simulink model "c00023M_harness"  (R2018a)
settings: Solver=ode3  StartTime=0.0  StopTime=10.0  RelTol=1e-3  EnableMultiTasking=on
undefined symbols (not defined in the file): b, DiscIntNeverNeededParam, J, K, L, PosMinimaW3, PosMinimaW4, R, sigbuilder_block
(part 22 of 72)

== system c00023M_harness/M154/S3 ==
  PhyMeasure : Inport
  SensorOut : Outport
  wires:
  PhyMeasure/1 -> SensorOut/1

== system c00023M_harness/M154/S4 ==
  PhyMeasure : Inport
  SensorOut : Outport
  wires:
  PhyMeasure/1 -> SensorOut/1

== system c00023M_harness/M155/Cyber ==
  note: Sensors
  note: Inputs For Window1
  note: Inputs for Window 2
  note: Inputs for window 3
  note: Inputs for window 4
  note: Users
  note: Users
  note: Sensors
  note: Users
  note: Sensors
  note: Users
  note: Sensors
  note: USERS
      | ---------------------------------
      | 0: None
      | 1: Ventana Arriba
      | 2: Ventana hasta arriba
      | 3: Ventana abajo
      | 4: Ventana hasta abajo
  note: 1: SUBE
      | 0: PARADO
      | -1 BAJA
  note: D = Driver (W1)
      | P1 = Passenger 1 (W2)
      | P2 = Passenger 2 (W3)
      | P3 = Passenger 3 (W4)
      | O = Obstacle
      | C = Control
      | Pri = Prioritizer
      | LD = LockDriver
      | PosW = PositionWindow
      | WL = WindowLogic
      | OW = ObstacleWindow
      | CWXC = ControlWindowXCentralized
      | S = Sensor
      | L = Lock
      | WPos = WindowPosition
      | M = Memory
      | InW = InputWindow
      | WIn = WindowInput
  PosW1 : Inport
  PosW2 : Inport  Port=2
  PosW3 : Inport  Port=3
  PosW4 : Inport  Port=4
  DW1 : Inport  Port=5
  DW3 : Inport  Port=6
  P1W2 : Inport  Port=7
  P2W3 : Inport  Port=8
  P3W4 : Inport  Port=9
  P1W4 : Inport  Port=10
  OW1 : Inport  Port=11
  OW2 : Inport  Port=12
  OW3 : Inport  Port=13
  OW4 : Inport  Port=14
  LD : Inport  Port=15
  CW3C : Inport  Port=16
  CW4C : Inport  Port=17
  Pri1 : Subsystem
  Pri4 : Subsystem
  WL : Subsystem
  WL1 : Subsystem
  WL2 : Subsystem
  WL3 : Subsystem
  W1 : Outport
  W2 : Outport  Port=2
  W3 : Outport  Port=3
  W4 : Outport  Port=4
  wires:
  CW4C/1 -> Pri4/3(CW4C)
  CW3C/1 -> Pri1/3(CW3C)
  WL3/1(WindowLogicOutput) -> W4/1
  WL2/1(WindowLogicOutput) -> W3/1
  Pri4/1(User) -> WL3/2(User)
  OW4/1 -> WL3/3(OW)
  PosW4/1 -> WL3/1(WPos)
  P1W4/1 -> Pri4/2(P1)
  P3W4/1 -> Pri4/1(P)
  P2W3/1 -> Pri1/2(P)
  DW3/1 -> Pri1/1(D)
  OW3/1 -> WL2/3(OW)
  PosW3/1 -> WL2/1(WPos)
  Pri1/1(User) -> WL2/2(User)
  WL1/1(WindowLogicOutput) -> W2/1
  OW2/1 -> WL1/3(OW)
  PosW2/1 -> WL1/1(WPos)
  WL/1(WindowLogicOutput) -> W1/1
  OW1/1 -> WL/3(OW)
  PosW1/1 -> WL/1(WPos)
  LD/1 -> WL2/4(L), WL3/4(L)
  DW1/1 -> WL/2(User)
  P1W2/1 -> WL1/2(User)

== system c00023M_harness/M155/Physical ==
  InW1 : Inport
  InW2 : Inport  Port=2
  InW3 : Inport  Port=3
  InW4 : Inport  Port=4
  W : Subsystem
  W5 : Subsystem
  W6 : Subsystem
  W7 : Subsystem
  W1 : Outport
  W2 : Outport  Port=2
  W3 : Outport  Port=3
  W4 : Outport  Port=4
  wires:
  W7/1(WPos) -> W4/1
  W6/1(WPos) -> W3/1
  W5/1(WPos) -> W2/1
  W/1(WPos) -> W1/1
  InW4/1 -> W7/1(WIn)
  InW3/1 -> W6/1(WIn)
  InW2/1 -> W5/1(WIn)
  InW1/1 -> W/1(WIn)

== system c00023M_harness/M155/S1 ==
  PhyMeasure : Inport
  SensorOut : Outport
  wires:
  PhyMeasure/1 -> SensorOut/1

== system c00023M_harness/M155/S2 ==
  PhyMeasure : Inport
  SensorOut : Outport
  wires:
  PhyMeasure/1 -> SensorOut/1

== system c00023M_harness/M155/S3 ==
  PhyMeasure : Inport
  SensorOut : Outport
  wires:
  PhyMeasure/1 -> SensorOut/1

== system c00023M_harness/M155/S4 ==
  PhyMeasure : Inport
  SensorOut : Outport
  wires:
  PhyMeasure/1 -> SensorOut/1

== system c00023M_harness/M156/Cyber ==
  note: Sensors
  note: Inputs For Window1
  note: Inputs for Window 2
  note: Inputs for window 3
  note: Inputs for window 4
  note: Users
  note: Users
  note: Sensors
  note: Users
  note: Sensors
  note: Users
  note: Sensors
  note: USERS
      | ---------------------------------
      | 0: None
      | 1: Ventana Arriba
      | 2: Ventana hasta arriba
      | 3: Ventana abajo
      | 4: Ventana hasta abajo
  note: 1: SUBE
      | 0: PARADO
      | -1 BAJA
  note: D = Driver (W1)
      | P1 = Passenger 1 (W2)
      | P2 = Passenger 2 (W3)
      | P3 = Passenger 3 (W4)
      | O = Obstacle
      | C = Control
      | Pri = Prioritizer
      | LD = LockDriver
      | PosW = PositionWindow
      | WL = WindowLogic
      | OW = ObstacleWindow
      | CWXC = ControlWindowXCentralized
      | S = Sensor
      | L = Lock
      | WPos = WindowPosition
      | M = Memory
      | InW = InputWindow
      | WIn = WindowInput
  PosW1 : Inport
  PosW2 : Inport  Port=2
  PosW3 : Inport  Port=3
  PosW4 : Inport  Port=4
  DW1 : Inport  Port=5
  DW3 : Inport  Port=6
  P1W2 : Inport  Port=7
  P2W3 : Inport  Port=8
  P3W4 : Inport  Port=9
  P1W4 : Inport  Port=10
  OW1 : Inport  Port=11
  OW2 : Inport  Port=12
  OW3 : Inport  Port=13
  OW4 : Inport  Port=14
  LD : Inport  Port=15
  CW3C : Inport  Port=16
  CW4C : Inport  Port=17
  Pri1 : Subsystem
  Pri4 : Subsystem
  WL : Subsystem
  WL1 : Subsystem
  WL2 : Subsystem
  WL3 : Subsystem
  W1 : Outport
  W2 : Outport  Port=2
  W3 : Outport  Port=3
  W4 : Outport  Port=4
  wires:
  CW4C/1 -> Pri4/3(CW4C)
  CW3C/1 -> Pri1/3(CW3C)
  WL3/1(WindowLogicOutput) -> W4/1
  WL2/1(WindowLogicOutput) -> W3/1
  Pri4/1(User) -> WL3/2(User)
  OW4/1 -> WL3/3(OW)
  PosW4/1 -> WL3/1(WPos)
  P1W4/1 -> Pri4/2(P1)
  P3W4/1 -> Pri4/1(P)
  P2W3/1 -> Pri1/2(P)
  DW3/1 -> Pri1/1(D)
  OW3/1 -> WL2/3(OW)
  PosW3/1 -> WL2/1(WPos)
  Pri1/1(User) -> WL2/2(User)
  WL1/1(WindowLogicOutput) -> W2/1
  OW2/1 -> WL1/3(OW)
  PosW2/1 -> WL1/1(WPos)
  WL/1(WindowLogicOutput) -> W1/1
  OW1/1 -> WL/3(OW)
  PosW1/1 -> WL/1(WPos)
  LD/1 -> WL2/4(L), WL3/4(L)
  DW1/1 -> WL/2(User)
  P1W2/1 -> WL1/2(User)

== system c00023M_harness/M156/Physical ==
  InW1 : Inport
  InW2 : Inport  Port=2
  InW3 : Inport  Port=3
  InW4 : Inport  Port=4
  W : Subsystem
  W5 : Subsystem
  W6 : Subsystem
  W7 : Subsystem
  W1 : Outport
  W2 : Outport  Port=2
  W3 : Outport  Port=3
  W4 : Outport  Port=4
  wires:
  W7/1(WPos) -> W4/1
  W6/1(WPos) -> W3/1
  W5/1(WPos) -> W2/1
  W/1(WPos) -> W1/1
  InW4/1 -> W7/1(WIn)
  InW3/1 -> W6/1(WIn)
  InW2/1 -> W5/1(WIn)
  InW1/1 -> W/1(WIn)

== system c00023M_harness/M156/S1 ==
  PhyMeasure : Inport
  SensorOut : Outport
  wires:
  PhyMeasure/1 -> SensorOut/1

== system c00023M_harness/M156/S2 ==
  PhyMeasure : Inport
  SensorOut : Outport
  wires:
  PhyMeasure/1 -> SensorOut/1

== system c00023M_harness/M156/S3 ==
  PhyMeasure : Inport
  SensorOut : Outport
  wires:
  PhyMeasure/1 -> SensorOut/1

== system c00023M_harness/M156/S4 ==
  PhyMeasure : Inport
  SensorOut : Outport
  wires:
  PhyMeasure/1 -> SensorOut/1

== system c00023M_harness/M157/Cyber ==
  note: Sensors
  note: Inputs For Window1
  note: Inputs for Window 2
  note: Inputs for window 3
  note: Inputs for window 4
  note: Users
  note: Users
  note: Sensors
  note: Users
  note: Sensors
  note: Users
  note: Sensors
  note: USERS
      | ---------------------------------
      | 0: None
      | 1: Ventana Arriba
      | 2: Ventana hasta arriba
      | 3: Ventana abajo
      | 4: Ventana hasta abajo
  note: 1: SUBE
      | 0: PARADO
      | -1 BAJA
  note: D = Driver (W1)
      | P1 = Passenger 1 (W2)
      | P2 = Passenger 2 (W3)
      | P3 = Passenger 3 (W4)
      | O = Obstacle
      | C = Control
      | Pri = Prioritizer
      | LD = LockDriver
      | PosW = PositionWindow
      | WL = WindowLogic
      | OW = ObstacleWindow
      | CWXC = ControlWindowXCentralized
      | S = Sensor
      | L = Lock
      | WPos = WindowPosition
      | M = Memory
      | InW = InputWindow
      | WIn = WindowInput
  PosW1 : Inport
  PosW2 : Inport  Port=2
  PosW3 : Inport  Port=3
  PosW4 : Inport  Port=4
  DW1 : Inport  Port=5
  DW3 : Inport  Port=6
  P1W2 : Inport  Port=7
  P2W3 : Inport  Port=8
  P3W4 : Inport  Port=9
  P1W4 : Inport  Port=10
  OW1 : Inport  Port=11
  OW2 : Inport  Port=12
  OW3 : Inport  Port=13
  OW4 : Inport  Port=14
  LD : Inport  Port=15
  CW3C : Inport  Port=16
  CW4C : Inport  Port=17
  Pri1 : Subsystem
  Pri4 : Subsystem
  WL : Subsystem
  WL1 : Subsystem
  WL2 : Subsystem
  WL3 : Subsystem
  W1 : Outport
  W2 : Outport  Port=2
  W3 : Outport  Port=3
  W4 : Outport  Port=4
  wires:
  CW4C/1 -> Pri4/3(CW4C)
  CW3C/1 -> Pri1/3(CW3C)
  WL3/1(WindowLogicOutput) -> W4/1
  WL2/1(WindowLogicOutput) -> W3/1
  Pri4/1(User) -> WL3/2(User)
  OW4/1 -> WL3/3(OW)
  PosW4/1 -> WL3/1(WPos)
  P1W4/1 -> Pri4/2(P1)
  P3W4/1 -> Pri4/1(P)
  P2W3/1 -> Pri1/2(P)
  DW3/1 -> Pri1/1(D)
  OW3/1 -> WL2/3(OW)
  PosW3/1 -> WL2/1(WPos)
  Pri1/1(User) -> WL2/2(User)
  WL1/1(WindowLogicOutput) -> W2/1
  OW2/1 -> WL1/3(OW)
  PosW2/1 -> WL1/1(WPos)
  WL/1(WindowLogicOutput) -> W1/1
  OW1/1 -> WL/3(OW)
  PosW1/1 -> WL/1(WPos)
  LD/1 -> WL2/4(L), WL3/4(L)
  DW1/1 -> WL/2(User)
  P1W2/1 -> WL1/2(User)

== system c00023M_harness/M157/Physical ==
  InW1 : Inport
  InW2 : Inport  Port=2
  InW3 : Inport  Port=3
  InW4 : Inport  Port=4
  W : Subsystem
  W5 : Subsystem
  W6 : Subsystem
  W7 : Subsystem
  W1 : Outport
  W2 : Outport  Port=2
  W3 : Outport  Port=3
  W4 : Outport  Port=4
  wires:
  W7/1(WPos) -> W4/1
  W6/1(WPos) -> W3/1
  W5/1(WPos) -> W2/1
  W/1(WPos) -> W1/1
  InW4/1 -> W7/1(WIn)
  InW3/1 -> W6/1(WIn)
  InW2/1 -> W5/1(WIn)
  InW1/1 -> W/1(WIn)

== system c00023M_harness/M157/S1 ==
  PhyMeasure : Inport
  SensorOut : Outport
  wires:
  PhyMeasure/1 -> SensorOut/1

== system c00023M_harness/M157/S2 ==
  PhyMeasure : Inport
  SensorOut : Outport
  wires:
  PhyMeasure/1 -> SensorOut/1

== system c00023M_harness/M157/S3 ==
  PhyMeasure : Inport
  SensorOut : Outport
  wires:
  PhyMeasure/1 -> SensorOut/1

== system c00023M_harness/M157/S4 ==
  PhyMeasure : Inport
  SensorOut : Outport
  wires:
  PhyMeasure/1 -> SensorOut/1

== system c00023M_harness/M158/Cyber ==
  note: Sensors
  note: Inputs For Window1
  note: Inputs for Window 2
  note: Inputs for window 3
  note: Inputs for window 4
  note: Users
  note: Users
  note: Sensors
  note: Users
  note: Sensors
  note: Users
  note: Sensors
  note: USERS
      | ---------------------------------
      | 0: None
      | 1: Ventana Arriba
      | 2: Ventana hasta arriba
      | 3: Ventana abajo
      | 4: Ventana hasta abajo
  note: 1: SUBE
      | 0: PARADO
      | -1 BAJA
  note: D = Driver (W1)
      | P1 = Passenger 1 (W2)
      | P2 = Passenger 2 (W3)
      | P3 = Passenger 3 (W4)
      | O = Obstacle
      | C = Control
      | Pri = Prioritizer
      | LD = LockDriver
      | PosW = PositionWindow
      | WL = WindowLogic
      | OW = ObstacleWindow
      | CWXC = ControlWindowXCentralized
      | S = Sensor
      | L = Lock
      | WPos = WindowPosition
      | M = Memory
      | InW = InputWindow
      | WIn = WindowInput
  PosW1 : Inport
  PosW2 : Inport  Port=2
  PosW3 : Inport  Port=3
  PosW4 : Inport  Port=4
  DW1 : Inport  Port=5
  DW3 : Inport  Port=6
  P1W2 : Inport  Port=7
  P2W3 : Inport  Port=8
  P3W4 : Inport  Port=9
  P1W4 : Inport  Port=10
  OW1 : Inport  Port=11
  OW2 : Inport  Port=12
  OW3 : Inport  Port=13
  OW4 : Inport  Port=14
  LD : Inport  Port=15
  CW3C : Inport  Port=16
  CW4C : Inport  Port=17
  Pri1 : Subsystem
  Pri4 : Subsystem
  WL : Subsystem
  WL1 : Subsystem
  WL2 : Subsystem
  WL3 : Subsystem
  W1 : Outport
  W2 : Outport  Port=2
  W3 : Outport  Port=3
  W4 : Outport  Port=4
  wires:
  CW4C/1 -> Pri4/3(CW4C)
  CW3C/1 -> Pri1/3(CW3C)
  WL3/1(WindowLogicOutput) -> W4/1
  WL2/1(WindowLogicOutput) -> W3/1
  Pri4/1(User) -> WL3/2(User)
  OW4/1 -> WL3/3(OW)
  PosW4/1 -> WL3/1(WPos)
  P1W4/1 -> Pri4/2(P1)
  P3W4/1 -> Pri4/1(P)
  P2W3/1 -> Pri1/2(P)
  DW3/1 -> Pri1/1(D)
  OW3/1 -> WL2/3(OW)
  PosW3/1 -> WL2/1(WPos)
  Pri1/1(User) -> WL2/2(User)
  WL1/1(WindowLogicOutput) -> W2/1
  OW2/1 -> WL1/3(OW)
  PosW2/1 -> WL1/1(WPos)
  WL/1(WindowLogicOutput) -> W1/1
  OW1/1 -> WL/3(OW)
  PosW1/1 -> WL/1(WPos)
  LD/1 -> WL2/4(L), WL3/4(L)
  DW1/1 -> WL/2(User)
  P1W2/1 -> WL1/2(User)

== system c00023M_harness/M158/Physical ==
  InW1 : Inport
  InW2 : Inport  Port=2
  InW3 : Inport  Port=3
  InW4 : Inport  Port=4
  W : Subsystem
  W5 : Subsystem
  W6 : Subsystem
  W7 : Subsystem
  W1 : Outport
  W2 : Outport  Port=2
  W3 : Outport  Port=3
  W4 : Outport  Port=4
  wires:
  W7/1(WPos) -> W4/1
  W6/1(WPos) -> W3/1
  W5/1(WPos) -> W2/1
  W/1(WPos) -> W1/1
  InW4/1 -> W7/1(WIn)
  InW3/1 -> W6/1(WIn)
  InW2/1 -> W5/1(WIn)
  InW1/1 -> W/1(WIn)

== system c00023M_harness/M158/S1 ==
  PhyMeasure : Inport
  SensorOut : Outport
  wires:
  PhyMeasure/1 -> SensorOut/1

== system c00023M_harness/M158/S2 ==
  PhyMeasure : Inport
  SensorOut : Outport
  wires:
  PhyMeasure/1 -> SensorOut/1

== system c00023M_harness/M158/S3 ==
  PhyMeasure : Inport
  SensorOut : Outport
  wires:
  PhyMeasure/1 -> SensorOut/1

== system c00023M_harness/M158/S4 ==
  PhyMeasure : Inport
  SensorOut : Outport
  wires:
  PhyMeasure/1 -> SensorOut/1

== system c00023M_harness/M159/Cyber ==
  note: Sensors
  note: Inputs For Window1
  note: Inputs for Window 2
  note: Inputs for window 3
  note: Inputs for window 4
  note: Users
  note: Users
  note: Sensors
  note: Users
  note: Sensors
  note: Users
  note: Sensors
  note: USERS
      | ---------------------------------
      | 0: None
      | 1: Ventana Arriba
      | 2: Ventana hasta arriba
      | 3: Ventana abajo
      | 4: Ventana hasta abajo
  note: 1: SUBE
      | 0: PARADO
      | -1 BAJA
  note: D = Driver (W1)
      | P1 = Passenger 1 (W2)
      | P2 = Passenger 2 (W3)
      | P3 = Passenger 3 (W4)
      | O = Obstacle
      | C = Control
      | Pri = Prioritizer
      | LD = LockDriver
      | PosW = PositionWindow
      | WL = WindowLogic
      | OW = ObstacleWindow
      | CWXC = ControlWindowXCentralized
      | S = Sensor
      | L = Lock
      | WPos = WindowPosition
      | M = Memory
      | InW = InputWindow
      | WIn = WindowInput
  PosW1 : Inport
  PosW2 : Inport  Port=2
  PosW3 : Inport  Port=3
  PosW4 : Inport  Port=4
  DW1 : Inport  Port=5
  DW3 : Inport  Port=6
  P1W2 : Inport  Port=7
  P2W3 : Inport  Port=8
  P3W4 : Inport  Port=9
  P1W4 : Inport  Port=10
  OW1 : Inport  Port=11
  OW2 : Inport  Port=12
  OW3 : Inport  Port=13
  OW4 : Inport  Port=14
  LD : Inport  Port=15
  CW3C : Inport  Port=16
  CW4C : Inport  Port=17
  Pri1 : Subsystem
  Pri4 : Subsystem
  WL : Subsystem
  WL1 : Subsystem
  WL2 : Subsystem
  WL3 : Subsystem
  W1 : Outport
  W2 : Outport  Port=2
  W3 : Outport  Port=3
  W4 : Outport  Port=4
  wires:
  CW4C/1 -> Pri4/3(CW4C)
  CW3C/1 -> Pri1/3(CW3C)
  WL3/1(WindowLogicOutput) -> W4/1
  WL2/1(WindowLogicOutput) -> W3/1
  Pri4/1(User) -> WL3/2(User)
  OW4/1 -> WL3/3(OW)
  PosW4/1 -> WL3/1(WPos)
  P1W4/1 -> Pri4/2(P1)
  P3W4/1 -> Pri4/1(P)
  P2W3/1 -> Pri1/2(P)
  DW3/1 -> Pri1/1(D)
  OW3/1 -> WL2/3(OW)
  PosW3/1 -> WL2/1(WPos)
  Pri1/1(User) -> WL2/2(User)
  WL1/1(WindowLogicOutput) -> W2/1
  OW2/1 -> WL1/3(OW)
  PosW2/1 -> WL1/1(WPos)
  WL/1(WindowLogicOutput) -> W1/1
  OW1/1 -> WL/3(OW)
  PosW1/1 -> WL/1(WPos)
  LD/1 -> WL2/4(L), WL3/4(L)
  DW1/1 -> WL/2(User)
  P1W2/1 -> WL1/2(User)

== system c00023M_harness/M159/Physical ==
  InW1 : Inport
  InW2 : Inport  Port=2
  InW3 : Inport  Port=3
  InW4 : Inport  Port=4
  W : Subsystem
  W5 : Subsystem
  W6 : Subsystem
  W7 : Subsystem
  W1 : Outport
  W2 : Outport  Port=2
  W3 : Outport  Port=3
  W4 : Outport  Port=4
  wires:
  W7/1(WPos) -> W4/1
  W6/1(WPos) -> W3/1
  W5/1(WPos) -> W2/1
  W/1(WPos) -> W1/1
  InW4/1 -> W7/1(WIn)
  InW3/1 -> W6/1(WIn)
  InW2/1 -> W5/1(WIn)
  InW1/1 -> W/1(WIn)

== system c00023M_harness/M159/S1 ==
  PhyMeasure : Inport
  SensorOut : Outport
  wires:
  PhyMeasure/1 -> SensorOut/1

== system c00023M_harness/M159/S2 ==
  PhyMeasure : Inport
  SensorOut : Outport
  wires:
  PhyMeasure/1 -> SensorOut/1

== system c00023M_harness/M159/S3 ==
  PhyMeasure : Inport
  SensorOut : Outport
  wires:
  PhyMeasure/1 -> SensorOut/1

== system c00023M_harness/M159/S4 ==
  PhyMeasure : Inport
  SensorOut : Outport
  wires:
  PhyMeasure/1 -> SensorOut/1

== system c00023M_harness/M160/Cyber ==
  note: Sensors
  note: Inputs For Window1
  note: Inputs for Window 2
  note: Inputs for window 3
  note: Inputs for window 4
  note: Users
  note: Users
  note: Sensors
  note: Users
  note: Sensors
  note: Users
  note: Sensors
  note: USERS
      | ---------------------------------
      | 0: None
      | 1: Ventana Arriba
      | 2: Ventana hasta arriba
      | 3: Ventana abajo
      | 4: Ventana hasta abajo
  note: 1: SUBE
      | 0: PARADO
      | -1 BAJA
  note: D = Driver (W1)
      | P1 = Passenger 1 (W2)
      | P2 = Passenger 2 (W3)
      | P3 = Passenger 3 (W4)
      | O = Obstacle
      | C = Control
      | Pri = Prioritizer
      | LD = LockDriver
      | PosW = PositionWindow
      | WL = WindowLogic
      | OW = ObstacleWindow
      | CWXC = ControlWindowXCentralized
      | S = Sensor
      | L = Lock
      | WPos = WindowPosition
      | M = Memory
      | InW = InputWindow
      | WIn = WindowInput
  PosW1 : Inport
  PosW2 : Inport  Port=2
  PosW3 : Inport  Port=3
  PosW4 : Inport  Port=4
  DW1 : Inport  Port=5
  DW3 : Inport  Port=6
  P1W2 : Inport  Port=7
  P2W3 : Inport  Port=8
  P3W4 : Inport  Port=9
  P1W4 : Inport  Port=10
  OW1 : Inport  Port=11
  OW2 : Inport  Port=12
  OW3 : Inport  Port=13
  OW4 : Inport  Port=14
  LD : Inport  Port=15
  CW3C : Inport  Port=16
  CW4C : Inport  Port=17
  Pri1 : Subsystem
  Pri4 : Subsystem
  WL : Subsystem
  WL1 : Subsystem
  WL2 : Subsystem
  WL3 : Subsystem
  W1 : Outport
  W2 : Outport  Port=2
  W3 : Outport  Port=3
  W4 : Outport  Port=4
  wires:
  CW4C/1 -> Pri4/3(CW4C)
  CW3C/1 -> Pri1/3(CW3C)
  WL3/1(WindowLogicOutput) -> W4/1
  WL2/1(WindowLogicOutput) -> W3/1
  Pri4/1(User) -> WL3/2(User)
  OW4/1 -> WL3/3(OW)
  PosW4/1 -> WL3/1(WPos)
  P1W4/1 -> Pri4/2(P1)
  P3W4/1 -> Pri4/1(P)
  P2W3/1 -> Pri1/2(P)
  DW3/1 -> Pri1/1(D)
  OW3/1 -> WL2/3(OW)
  PosW3/1 -> WL2/1(WPos)
  Pri1/1(User) -> WL2/2(User)
  WL1/1(WindowLogicOutput) -> W2/1
  OW2/1 -> WL1/3(OW)
  PosW2/1 -> WL1/1(WPos)
  WL/1(WindowLogicOutput) -> W1/1
  OW1/1 -> WL/3(OW)
  PosW1/1 -> WL/1(WPos)
  LD/1 -> WL2/4(L), WL3/4(L)
  DW1/1 -> WL/2(User)
  P1W2/1 -> WL1/2(User)

== system c00023M_harness/M160/Physical ==
  InW1 : Inport
  InW2 : Inport  Port=2
  InW3 : Inport  Port=3
  InW4 : Inport  Port=4
  W : Subsystem
  W5 : Subsystem
  W6 : Subsystem
  W7 : Subsystem
  W1 : Outport
  W2 : Outport  Port=2
  W3 : Outport  Port=3
  W4 : Outport  Port=4
  wires:
  W7/1(WPos) -> W4/1
  W6/1(WPos) -> W3/1
  W5/1(WPos) -> W2/1
  W/1(WPos) -> W1/1
  InW4/1 -> W7/1(WIn)
  InW3/1 -> W6/1(WIn)
  InW2/1 -> W5/1(WIn)
  InW1/1 -> W/1(WIn)

== system c00023M_harness/M160/S1 ==
  PhyMeasure : Inport
  SensorOut : Outport
  wires:
  PhyMeasure/1 -> SensorOut/1

== system c00023M_harness/M160/S2 ==
  PhyMeasure : Inport
  SensorOut : Outport
  wires:
  PhyMeasure/1 -> SensorOut/1

== system c00023M_harness/M160/S3 ==
  PhyMeasure : Inport
  SensorOut : Outport
  wires:
  PhyMeasure/1 -> SensorOut/1

== system c00023M_harness/M160/S4 ==
  PhyMeasure : Inport
  SensorOut : Outport
  wires:
  PhyMeasure/1 -> SensorOut/1

== system c00023M_harness/M161/Cyber ==
  note: Sensors
  note: Inputs For Window1
  note: Inputs for Window 2
  note: Inputs for window 3
  note: Inputs for window 4
  note: Users
  note: Users
  note: Sensors
  note: Users
  note: Sensors
  note: Users
  note: Sensors
  note: USERS
      | ---------------------------------
      | 0: None
      | 1: Ventana Arriba
      | 2: Ventana hasta arriba
      | 3: Ventana abajo
      | 4: Ventana hasta abajo
  note: 1: SUBE
      | 0: PARADO
      | -1 BAJA
  note: D = Driver (W1)
      | P1 = Passenger 1 (W2)
      | P2 = Passenger 2 (W3)
      | P3 = Passenger 3 (W4)
      | O = Obstacle
      | C = Control
      | Pri = Prioritizer
      | LD = LockDriver
      | PosW = PositionWindow
      | WL = WindowLogic
      | OW = ObstacleWindow
      | CWXC = ControlWindowXCentralized
      | S = Sensor
      | L = Lock
      | WPos = WindowPosition
      | M = Memory
      | InW = InputWindow
      | WIn = WindowInput
  PosW1 : Inport
  PosW2 : Inport  Port=2
  PosW3 : Inport  Port=3
  PosW4 : Inport  Port=4
  DW1 : Inport  Port=5
  DW3 : Inport  Port=6
  P1W2 : Inport  Port=7
  P2W3 : Inport  Port=8
  P3W4 : Inport  Port=9
  P1W4 : Inport  Port=10
  OW1 : Inport  Port=11
  OW2 : Inport  Port=12
  OW3 : Inport  Port=13
  OW4 : Inport  Port=14
  LD : Inport  Port=15
  CW3C : Inport  Port=16
  CW4C : Inport  Port=17
  Pri1 : Subsystem
  Pri4 : Subsystem
  WL : Subsystem
  WL1 : Subsystem
  WL2 : Subsystem
  WL3 : Subsystem
  W1 : Outport
  W2 : Outport  Port=2
  W3 : Outport  Port=3
  W4 : Outport  Port=4
  wires:
  CW4C/1 -> Pri4/3(CW4C)
  CW3C/1 -> Pri1/3(CW3C)
  WL3/1(WindowLogicOutput) -> W4/1
  WL2/1(WindowLogicOutput) -> W3/1
  Pri4/1(User) -> WL3/2(User)
  OW4/1 -> WL3/3(OW)
  PosW4/1 -> WL3/1(WPos)
  P1W4/1 -> Pri4/2(P1)
  P3W4/1 -> Pri4/1(P)
  P2W3/1 -> Pri1/2(P)
  DW3/1 -> Pri1/1(D)
  OW3/1 -> WL2/3(OW)
  PosW3/1 -> WL2/1(WPos)
  Pri1/1(User) -> WL2/2(User)
  WL1/1(WindowLogicOutput) -> W2/1
  OW2/1 -> WL1/3(OW)
  PosW2/1 -> WL1/1(WPos)
  WL/1(WindowLogicOutput) -> W1/1
  OW1/1 -> WL/3(OW)
  PosW1/1 -> WL/1(WPos)
  LD/1 -> WL2/4(L), WL3/4(L)
  DW1/1 -> WL/2(User)
  P1W2/1 -> WL1/2(User)

== system c00023M_harness/M161/Physical ==
  InW1 : Inport
  InW2 : Inport  Port=2
  InW3 : Inport  Port=3
  InW4 : Inport  Port=4
  W : Subsystem
  W5 : Subsystem
  W6 : Subsystem
  W7 : Subsystem
  W1 : Outport
  W2 : Outport  Port=2
  W3 : Outport  Port=3
  W4 : Outport  Port=4
  wires:
  W7/1(WPos) -> W4/1
  W6/1(WPos) -> W3/1
  W5/1(WPos) -> W2/1
  W/1(WPos) -> W1/1
  InW4/1 -> W7/1(WIn)
  InW3/1 -> W6/1(WIn)
  InW2/1 -> W5/1(WIn)
  InW1/1 -> W/1(WIn)

== system c00023M_harness/M161/S1 ==
  PhyMeasure : Inport
  SensorOut : Outport
  wires:
  PhyMeasure/1 -> SensorOut/1

== system c00023M_harness/M161/S2 ==
  PhyMeasure : Inport
  SensorOut : Outport
  wires:
  PhyMeasure/1 -> SensorOut/1

== system c00023M_harness/M161/S3 ==
  PhyMeasure : Inport
  SensorOut : Outport
  wires:
  PhyMeasure/1 -> SensorOut/1

== system c00023M_harness/M161/S4 ==
  PhyMeasure : Inport
  SensorOut : Outport
  wires:
  PhyMeasure/1 -> SensorOut/1

== system c00023M_harness/M162/Cyber ==
  note: Sensors
  note: Inputs For Window1
  note: Inputs for Window 2
  note: Inputs for window 3
  note: Inputs for window 4
  note: Users
  note: Users
  note: Sensors
  note: Users
  note: Sensors
  note: Users
  note: Sensors
  note: USERS
      | ---------------------------------
      | 0: None
      | 1: Ventana Arriba
      | 2: Ventana hasta arriba
      | 3: Ventana abajo
      | 4: Ventana hasta abajo
  note: 1: SUBE
      | 0: PARADO
      | -1 BAJA
  note: D = Driver (W1)
      | P1 = Passenger 1 (W2)
      | P2 = Passenger 2 (W3)
      | P3 = Passenger 3 (W4)
      | O = Obstacle
      | C = Control
      | Pri = Prioritizer
      | LD = LockDriver
      | PosW = PositionWindow
      | WL = WindowLogic
      | OW = ObstacleWindow
      | CWXC = ControlWindowXCentralized
      | S = Sensor
      | L = Lock
      | WPos = WindowPosition
      | M = Memory
      | InW = InputWindow
      | WIn = WindowInput
  PosW1 : Inport
  PosW2 : Inport  Port=2
  PosW3 : Inport  Port=3
  PosW4 : Inport  Port=4
  DW1 : Inport  Port=5
  DW3 : Inport  Port=6
  P1W2 : Inport  Port=7
  P2W3 : Inport  Port=8
  P3W4 : Inport  Port=9
  P1W4 : Inport  Port=10
  OW1 : Inport  Port=11
  OW2 : Inport  Port=12
  OW3 : Inport  Port=13
  OW4 : Inport  Port=14
  LD : Inport  Port=15
  CW3C : Inport  Port=16
  CW4C : Inport  Port=17
  Pri1 : Subsystem
  Pri4 : Subsystem
  WL : Subsystem
  WL1 : Subsystem
  WL2 : Subsystem
  WL3 : Subsystem
  W1 : Outport
  W2 : Outport  Port=2
  W3 : Outport  Port=3
  W4 : Outport  Port=4
  wires:
  CW4C/1 -> Pri4/3(CW4C)
  CW3C/1 -> Pri1/3(CW3C)
  WL3/1(WindowLogicOutput) -> W4/1
  WL2/1(WindowLogicOutput) -> W3/1
  Pri4/1(User) -> WL3/2(User)
  OW4/1 -> WL3/3(OW)
  PosW4/1 -> WL3/1(WPos)
  P1W4/1 -> Pri4/2(P1)
  P3W4/1 -> Pri4/1(P)
  P2W3/1 -> Pri1/2(P)
  DW3/1 -> Pri1/1(D)
  OW3/1 -> WL2/3(OW)
  PosW3/1 -> WL2/1(WPos)
  Pri1/1(User) -> WL2/2(User)
  WL1/1(WindowLogicOutput) -> W2/1
  OW2/1 -> WL1/3(OW)
  PosW2/1 -> WL1/1(WPos)
  WL/1(WindowLogicOutput) -> W1/1
  OW1/1 -> WL/3(OW)
  PosW1/1 -> WL/1(WPos)
  LD/1 -> WL2/4(L), WL3/4(L)
  DW1/1 -> WL/2(User)
  P1W2/1 -> WL1/2(User)

== system c00023M_harness/M162/Physical ==
  InW1 : Inport
  InW2 : Inport  Port=2
  InW3 : Inport  Port=3
  InW4 : Inport  Port=4
  W : Subsystem
  W5 : Subsystem
  W6 : Subsystem
  W7 : Subsystem
  W1 : Outport
  W2 : Outport  Port=2
  W3 : Outport  Port=3
  W4 : Outport  Port=4
  wires:
  W7/1(WPos) -> W4/1
  W6/1(WPos) -> W3/1
  W5/1(WPos) -> W2/1
  W/1(WPos) -> W1/1
  InW4/1 -> W7/1(WIn)
  InW3/1 -> W6/1(WIn)
  InW2/1 -> W5/1(WIn)
  InW1/1 -> W/1(WIn)

== system c00023M_harness/M162/S1 ==
  PhyMeasure : Inport
  SensorOut : Outport
  wires:
  PhyMeasure/1 -> SensorOut/1

== system c00023M_harness/M162/S2 ==
  PhyMeasure : Inport
  SensorOut : Outport
  wires:
  PhyMeasure/1 -> SensorOut/1

== system c00023M_harness/M162/S3 ==
  PhyMeasure : Inport
  SensorOut : Outport
  wires:
  PhyMeasure/1 -> SensorOut/1

== system c00023M_harness/M162/S4 ==
  PhyMeasure : Inport
  SensorOut : Outport
  wires:
  PhyMeasure/1 -> SensorOut/1

== system c00023M_harness/M163/Cyber ==
  note: Sensors
  note: Inputs For Window1
  note: Inputs for Window 2
  note: Inputs for window 3
  note: Inputs for window 4
  note: Users
  note: Users
  note: Sensors
  note: Users
  note: Sensors
  note: Users
  note: Sensors
  note: USERS
      | ---------------------------------
      | 0: None
      | 1: Ventana Arriba
      | 2: Ventana hasta arriba
      | 3: Ventana abajo
      | 4: Ventana hasta abajo
  note: 1: SUBE
      | 0: PARADO
      | -1 BAJA
  note: D = Driver (W1)
      | P1 = Passenger 1 (W2)
      | P2 = Passenger 2 (W3)
      | P3 = Passenger 3 (W4)
      | O = Obstacle
      | C = Control
      | Pri = Prioritizer
      | LD = LockDriver
      | PosW = PositionWindow
      | WL = WindowLogic
      | OW = ObstacleWindow
      | CWXC = ControlWindowXCentralized
      | S = Sensor
      | L = Lock
      | WPos = WindowPosition
      | M = Memory
      | InW = InputWindow
      | WIn = WindowInput
  PosW1 : Inport
  PosW2 : Inport  Port=2
  PosW3 : Inport  Port=3
  PosW4 : Inport  Port=4
  DW1 : Inport  Port=5
  DW3 : Inport  Port=6
  P1W2 : Inport  Port=7
  P2W3 : Inport  Port=8
  P3W4 : Inport  Port=9
  P1W4 : Inport  Port=10
  OW1 : Inport  Port=11
  OW2 : Inport  Port=12
  OW3 : Inport  Port=13
  OW4 : Inport  Port=14
  LD : Inport  Port=15
  CW3C : Inport  Port=16
  CW4C : Inport  Port=17
  Pri1 : Subsystem
  Pri4 : Subsystem
  WL : Subsystem
  WL1 : Subsystem
  WL2 : Subsystem
  WL3 : Subsystem
  W1 : Outport
  W2 : Outport  Port=2
  W3 : Outport  Port=3
  W4 : Outport  Port=4
  wires:
  CW4C/1 -> Pri4/3(CW4C)
  CW3C/1 -> Pri1/3(CW3C)
  WL3/1(WindowLogicOutput) -> W4/1
  WL2/1(WindowLogicOutput) -> W3/1
  Pri4/1(User) -> WL3/2(User)
  OW4/1 -> WL3/3(OW)
  PosW4/1 -> WL3/1(WPos)
  P1W4/1 -> Pri4/2(P1)
  P3W4/1 -> Pri4/1(P)
  P2W3/1 -> Pri1/2(P)
  DW3/1 -> Pri1/1(D)
  OW3/1 -> WL2/3(OW)
  PosW3/1 -> WL2/1(WPos)
  Pri1/1(User) -> WL2/2(User)
  WL1/1(WindowLogicOutput) -> W2/1
  OW2/1 -> WL1/3(OW)
  PosW2/1 -> WL1/1(WPos)
  WL/1(WindowLogicOutput) -> W1/1
  OW1/1 -> WL/3(OW)
  PosW1/1 -> WL/1(WPos)
  LD/1 -> WL2/4(L), WL3/4(L)
  DW1/1 -> WL/2(User)
  P1W2/1 -> WL1/2(User)

== system c00023M_harness/M163/Physical ==
  InW1 : Inport
  InW2 : Inport  Port=2
  InW3 : Inport  Port=3
  InW4 : Inport  Port=4
  W : Subsystem
  W5 : Subsystem
  W6 : Subsystem
  W7 : Subsystem
  W1 : Outport
  W2 : Outport  Port=2
  W3 : Outport  Port=3
  W4 : Outport  Port=4
  wires:
  W7/1(WPos) -> W4/1
  W6/1(WPos) -> W3/1
  W5/1(WPos) -> W2/1
  W/1(WPos) -> W1/1
  InW4/1 -> W7/1(WIn)
  InW3/1 -> W6/1(WIn)
  InW2/1 -> W5/1(WIn)
  InW1/1 -> W/1(WIn)

== system c00023M_harness/M163/S1 ==
  PhyMeasure : Inport
  SensorOut : Outport
  wires:
  PhyMeasure/1 -> SensorOut/1

== system c00023M_harness/M163/S2 ==
  PhyMeasure : Inport
  SensorOut : Outport
  wires:
  PhyMeasure/1 -> SensorOut/1

== system c00023M_harness/M163/S3 ==
  PhyMeasure : Inport
  SensorOut : Outport
  wires:
  PhyMeasure/1 -> SensorOut/1

== system c00023M_harness/M163/S4 ==
  PhyMeasure : Inport
  SensorOut : Outport
  wires:
  PhyMeasure/1 -> SensorOut/1

== system c00023M_harness/M164/Cyber ==
  note: Sensors
  note: Inputs For Window1
  note: Inputs for Window 2
  note: Inputs for window 3
  note: Inputs for window 4
  note: Users
  note: Users
  note: Sensors
  note: Users
  note: Sensors
  note: Users
  note: Sensors
  note: USERS
      | ---------------------------------
      | 0: None
      | 1: Ventana Arriba
      | 2: Ventana hasta arriba
      | 3: Ventana abajo
      | 4: Ventana hasta abajo
  note: 1: SUBE
      | 0: PARADO
      | -1 BAJA
  note: D = Driver (W1)
      | P1 = Passenger 1 (W2)
      | P2 = Passenger 2 (W3)
      | P3 = Passenger 3 (W4)
      | O = Obstacle
      | C = Control
      | Pri = Prioritizer
      | LD = LockDriver
      | PosW = PositionWindow
      | WL = WindowLogic
      | OW = ObstacleWindow
      | CWXC = ControlWindowXCentralized
      | S = Sensor
      | L = Lock
      | WPos = WindowPosition
      | M = Memory
      | InW = InputWindow
      | WIn = WindowInput
  PosW1 : Inport
  PosW2 : Inport  Port=2
  PosW3 : Inport  Port=3
  PosW4 : Inport  Port=4
  DW1 : Inport  Port=5
  DW3 : Inport  Port=6
  P1W2 : Inport  Port=7
  P2W3 : Inport  Port=8
  P3W4 : Inport  Port=9
  P1W4 : Inport  Port=10
  OW1 : Inport  Port=11
  OW2 : Inport  Port=12
  OW3 : Inport  Port=13
  OW4 : Inport  Port=14
  LD : Inport  Port=15
  CW3C : Inport  Port=16
  CW4C : Inport  Port=17
  Pri1 : Subsystem
  Pri4 : Subsystem
  WL : Subsystem
  WL1 : Subsystem
  WL2 : Subsystem
  WL3 : Subsystem
  W1 : Outport
  W2 : Outport  Port=2
  W3 : Outport  Port=3
  W4 : Outport  Port=4
  wires:
  CW4C/1 -> Pri4/3(CW4C)
  CW3C/1 -> Pri1/3(CW3C)
  WL3/1(WindowLogicOutput) -> W4/1
  WL2/1(WindowLogicOutput) -> W3/1
  Pri4/1(User) -> WL3/2(User)
  OW4/1 -> WL3/3(OW)
  PosW4/1 -> WL3/1(WPos)
  P1W4/1 -> Pri4/2(P1)
  P3W4/1 -> Pri4/1(P)
  P2W3/1 -> Pri1/2(P)
  DW3/1 -> Pri1/1(D)
  OW3/1 -> WL2/3(OW)
  PosW3/1 -> WL2/1(WPos)
  Pri1/1(User) -> WL2/2(User)
  WL1/1(WindowLogicOutput) -> W2/1
  OW2/1 -> WL1/3(OW)
  PosW2/1 -> WL1/1(WPos)
  WL/1(WindowLogicOutput) -> W1/1
  OW1/1 -> WL/3(OW)
  PosW1/1 -> WL/1(WPos)
  LD/1 -> WL2/4(L), WL3/4(L)
  DW1/1 -> WL/2(User)
  P1W2/1 -> WL1/2(User)

== system c00023M_harness/M164/Physical ==
  InW1 : Inport
  InW2 : Inport  Port=2
  InW3 : Inport  Port=3
  InW4 : Inport  Port=4
  W : Subsystem
  W5 : Subsystem
  W6 : Subsystem
  W7 : Subsystem
  W1 : Outport
  W2 : Outport  Port=2
  W3 : Outport  Port=3
  W4 : Outport  Port=4
  wires:
  W7/1(WPos) -> W4/1
  W6/1(WPos) -> W3/1
  W5/1(WPos) -> W2/1
  W/1(WPos) -> W1/1
  InW4/1 -> W7/1(WIn)
  InW3/1 -> W6/1(WIn)
  InW2/1 -> W5/1(WIn)
  InW1/1 -> W/1(WIn)

== system c00023M_harness/M164/S1 ==
  PhyMeasure : Inport
  SensorOut : Outport
  wires:
  PhyMeasure/1 -> SensorOut/1

== system c00023M_harness/M164/S2 ==
  PhyMeasure : Inport
  SensorOut : Outport
  wires:
  PhyMeasure/1 -> SensorOut/1

== system c00023M_harness/M164/S3 ==
  PhyMeasure : Inport
  SensorOut : Outport
  wires:
  PhyMeasure/1 -> SensorOut/1

== system c00023M_harness/M164/S4 ==
  PhyMeasure : Inport
  SensorOut : Outport
  wires:
  PhyMeasure/1 -> SensorOut/1

== system c00023M_harness/M165/Cyber ==
  note: Sensors
  note: Inputs For Window1
  note: Inputs for Window 2
  note: Inputs for window 3
  note: Inputs for window 4
  note: Users
  note: Users
  note: Sensors
  note: Users
  note: Sensors
  note: Users
  note: Sensors
  note: USERS
      | ---------------------------------
      | 0: None
      | 1: Ventana Arriba
      | 2: Ventana hasta arriba
      | 3: Ventana abajo
      | 4: Ventana hasta abajo
  note: 1: SUBE
      | 0: PARADO
      | -1 BAJA
  note: D = Driver (W1)
      | P1 = Passenger 1 (W2)
      | P2 = Passenger 2 (W3)
      | P3 = Passenger 3 (W4)
      | O = Obstacle
      | C = Control
      | Pri = Prioritizer
      | LD = LockDriver
      | PosW = PositionWindow
      | WL = WindowLogic
      | OW = ObstacleWindow
      | CWXC = ControlWindowXCentralized
      | S = Sensor
      | L = Lock
      | WPos = WindowPosition
      | M = Memory
      | InW = InputWindow
      | WIn = WindowInput
  PosW1 : Inport
  PosW2 : Inport  Port=2
  PosW3 : Inport  Port=3
  PosW4 : Inport  Port=4
  DW1 : Inport  Port=5
  DW3 : Inport  Port=6
  P1W2 : Inport  Port=7
  P2W3 : Inport  Port=8
  P3W4 : Inport  Port=9
  P1W4 : Inport  Port=10
  OW1 : Inport  Port=11
  OW2 : Inport  Port=12
  OW3 : Inport  Port=13
  OW4 : Inport  Port=14
  LD : Inport  Port=15
  CW3C : Inport  Port=16
  CW4C : Inport  Port=17
  Pri1 : Subsystem
  Pri4 : Subsystem
  WL : Subsystem
  WL1 : Subsystem
  WL2 : Subsystem
  WL3 : Subsystem
  W1 : Outport
  W2 : Outport  Port=2
  W3 : Outport  Port=3
  W4 : Outport  Port=4
  wires:
  CW4C/1 -> Pri4/3(CW4C)
  CW3C/1 -> Pri1/3(CW3C)
  WL3/1(WindowLogicOutput) -> W4/1
  WL2/1(WindowLogicOutput) -> W3/1
  Pri4/1(User) -> WL3/2(User)
  OW4/1 -> WL3/3(OW)
  PosW4/1 -> WL3/1(WPos)
  P1W4/1 -> Pri4/2(P1)
  P3W4/1 -> Pri4/1(P)
  P2W3/1 -> Pri1/2(P)
  DW3/1 -> Pri1/1(D)
  OW3/1 -> WL2/3(OW)
  PosW3/1 -> WL2/1(WPos)
  Pri1/1(User) -> WL2/2(User)
  WL1/1(WindowLogicOutput) -> W2/1
  OW2/1 -> WL1/3(OW)
  PosW2/1 -> WL1/1(WPos)
  WL/1(WindowLogicOutput) -> W1/1
  OW1/1 -> WL/3(OW)
  PosW1/1 -> WL/1(WPos)
  LD/1 -> WL2/4(L), WL3/4(L)
  DW1/1 -> WL/2(User)
  P1W2/1 -> WL1/2(User)

== system c00023M_harness/M165/Physical ==
  InW1 : Inport
  InW2 : Inport  Port=2
  InW3 : Inport  Port=3
  InW4 : Inport  Port=4
  W : Subsystem
  W5 : Subsystem
  W6 : Subsystem
  W7 : Subsystem
  W1 : Outport
  W2 : Outport  Port=2
  W3 : Outport  Port=3
  W4 : Outport  Port=4
  wires:
  W7/1(WPos) -> W4/1
  W6/1(WPos) -> W3/1
  W5/1(WPos) -> W2/1
  W/1(WPos) -> W1/1
  InW4/1 -> W7/1(WIn)
  InW3/1 -> W6/1(WIn)
  InW2/1 -> W5/1(WIn)
  InW1/1 -> W/1(WIn)

== system c00023M_harness/M165/S1 ==
  PhyMeasure : Inport
  SensorOut : Outport
  wires:
  PhyMeasure/1 -> SensorOut/1

== system c00023M_harness/M165/S2 ==
  PhyMeasure : Inport
  SensorOut : Outport
  wires:
  PhyMeasure/1 -> SensorOut/1

== system c00023M_harness/M165/S3 ==
  PhyMeasure : Inport
  SensorOut : Outport
  wires:
  PhyMeasure/1 -> SensorOut/1

== system c00023M_harness/M165/S4 ==
  PhyMeasure : Inport
  SensorOut : Outport
  wires:
  PhyMeasure/1 -> SensorOut/1

== system c00023M_harness/M166/Cyber ==
  note: Sensors
  note: Inputs For Window1
  note: Inputs for Window 2
  note: Inputs for window 3
  note: Inputs for window 4
  note: Users
  note: Users
  note: Sensors
  note: Users
  note: Sensors
  note: Users
  note: Sensors
  note: USERS
      | ---------------------------------
      | 0: None
      | 1: Ventana Arriba
      | 2: Ventana hasta arriba
      | 3: Ventana abajo
      | 4: Ventana hasta abajo
  note: 1: SUBE
      | 0: PARADO
      | -1 BAJA
  note: D = Driver (W1)
      | P1 = Passenger 1 (W2)
      | P2 = Passenger 2 (W3)
      | P3 = Passenger 3 (W4)
      | O = Obstacle
      | C = Control
      | Pri = Prioritizer
      | LD = LockDriver
      | PosW = PositionWindow
      | WL = WindowLogic
      | OW = ObstacleWindow
      | CWXC = ControlWindowXCentralized
      | S = Sensor
      | L = Lock
      | WPos = WindowPosition
      | M = Memory
      | InW = InputWindow
      | WIn = WindowInput
  PosW1 : Inport
  PosW2 : Inport  Port=2
  PosW3 : Inport  Port=3
  PosW4 : Inport  Port=4
  DW1 : Inport  Port=5
  DW3 : Inport  Port=6
  P1W2 : Inport  Port=7
  P2W3 : Inport  Port=8
  P3W4 : Inport  Port=9
  P1W4 : Inport  Port=10
  OW1 : Inport  Port=11
  OW2 : Inport  Port=12
  OW3 : Inport  Port=13
  OW4 : Inport  Port=14
  LD : Inport  Port=15
  CW3C : Inport  Port=16
  CW4C : Inport  Port=17
  Pri1 : Subsystem
  Pri4 : Subsystem
  WL : Subsystem
  WL1 : Subsystem
  WL2 : Subsystem
  WL3 : Subsystem
  W1 : Outport
  W2 : Outport  Port=2
  W3 : Outport  Port=3
  W4 : Outport  Port=4
  wires:
  CW4C/1 -> Pri4/3(CW4C)
  CW3C/1 -> Pri1/3(CW3C)
  WL3/1(WindowLogicOutput) -> W4/1
  WL2/1(WindowLogicOutput) -> W3/1
  Pri4/1(User) -> WL3/2(User)
  OW4/1 -> WL3/3(OW)
  PosW4/1 -> WL3/1(WPos)
  P1W4/1 -> Pri4/2(P1)
  P3W4/1 -> Pri4/1(P)
  P2W3/1 -> Pri1/2(P)
  DW3/1 -> Pri1/1(D)
  OW3/1 -> WL2/3(OW)
  PosW3/1 -> WL2/1(WPos)
  Pri1/1(User) -> WL2/2(User)
  WL1/1(WindowLogicOutput) -> W2/1
  OW2/1 -> WL1/3(OW)
  PosW2/1 -> WL1/1(WPos)
  WL/1(WindowLogicOutput) -> W1/1
  OW1/1 -> WL/3(OW)
  PosW1/1 -> WL/1(WPos)
  LD/1 -> WL2/4(L), WL3/4(L)
  DW1/1 -> WL/2(User)
  P1W2/1 -> WL1/2(User)

== system c00023M_harness/M166/Physical ==
  InW1 : Inport
  InW2 : Inport  Port=2
  InW3 : Inport  Port=3
  InW4 : Inport  Port=4
  W : Subsystem
  W5 : Subsystem
  W6 : Subsystem
  W7 : Subsystem
  W1 : Outport
  W2 : Outport  Port=2
  W3 : Outport  Port=3
  W4 : Outport  Port=4
  wires:
  W7/1(WPos) -> W4/1
  W6/1(WPos) -> W3/1
  W5/1(WPos) -> W2/1
  W/1(WPos) -> W1/1
  InW4/1 -> W7/1(WIn)
  InW3/1 -> W6/1(WIn)
  InW2/1 -> W5/1(WIn)
  InW1/1 -> W/1(WIn)

== system c00023M_harness/M166/S1 ==
  PhyMeasure : Inport
  SensorOut : Outport
  wires:
  PhyMeasure/1 -> SensorOut/1

== system c00023M_harness/M166/S2 ==
  PhyMeasure : Inport
  SensorOut : Outport
  wires:
  PhyMeasure/1 -> SensorOut/1

== system c00023M_harness/M166/S3 ==
  PhyMeasure : Inport
  SensorOut : Outport
  wires:
  PhyMeasure/1 -> SensorOut/1

== system c00023M_harness/M166/S4 ==
  PhyMeasure : Inport
  SensorOut : Outport
  wires:
  PhyMeasure/1 -> SensorOut/1

== system c00023M_harness/M167/Cyber ==
  note: Sensors
  note: Inputs For Window1
  note: Inputs for Window 2
  note: Inputs for window 3
  note: Inputs for window 4
  note: Users
  note: Users
  note: Sensors
  note: Users
  note: Sensors
  note: Users
  note: Sensors
  note: USERS
      | ---------------------------------
      | 0: None
      | 1: Ventana Arriba
      | 2: Ventana hasta arriba
      | 3: Ventana abajo
      | 4: Ventana hasta abajo
  note: 1: SUBE
      | 0: PARADO
      | -1 BAJA
  note: D = Driver (W1)
      | P1 = Passenger 1 (W2)
      | P2 = Passenger 2 (W3)
      | P3 = Passenger 3 (W4)
      | O = Obstacle
      | C = Control
      | Pri = Prioritizer
      | LD = LockDriver
      | PosW = PositionWindow
      | WL = WindowLogic
      | OW = ObstacleWindow
      | CWXC = ControlWindowXCentralized
      | S = Sensor
      | L = Lock
      | WPos = WindowPosition
      | M = Memory
      | InW = InputWindow
      | WIn = WindowInput
  PosW1 : Inport
  PosW2 : Inport  Port=2
  PosW3 : Inport  Port=3
  PosW4 : Inport  Port=4
  DW1 : Inport  Port=5
  DW3 : Inport  Port=6
  P1W2 : Inport  Port=7
  P2W3 : Inport  Port=8
  P3W4 : Inport  Port=9
  P1W4 : Inport  Port=10
  OW1 : Inport  Port=11
  OW2 : Inport  Port=12
  OW3 : Inport  Port=13
  OW4 : Inport  Port=14
  LD : Inport  Port=15
  CW3C : Inport  Port=16
  CW4C : Inport  Port=17
  Pri1 : Subsystem
  Pri4 : Subsystem
  WL : Subsystem
  WL1 : Subsystem
  WL2 : Subsystem
  WL3 : Subsystem
  W1 : Outport
  W2 : Outport  Port=2
  W3 : Outport  Port=3
  W4 : Outport  Port=4
  wires:
  CW4C/1 -> Pri4/3(CW4C)
  CW3C/1 -> Pri1/3(CW3C)
  WL3/1(WindowLogicOutput) -> W4/1
  WL2/1(WindowLogicOutput) -> W3/1
  Pri4/1(User) -> WL3/2(User)
  OW4/1 -> WL3/3(OW)
  PosW4/1 -> WL3/1(WPos)
  P1W4/1 -> Pri4/2(P1)
  P3W4/1 -> Pri4/1(P)
  P2W3/1 -> Pri1/2(P)
  DW3/1 -> Pri1/1(D)
  OW3/1 -> WL2/3(OW)
  PosW3/1 -> WL2/1(WPos)
  Pri1/1(User) -> WL2/2(User)
  WL1/1(WindowLogicOutput) -> W2/1
  OW2/1 -> WL1/3(OW)
  PosW2/1 -> WL1/1(WPos)
  WL/1(WindowLogicOutput) -> W1/1
  OW1/1 -> WL/3(OW)
  PosW1/1 -> WL/1(WPos)
  LD/1 -> WL2/4(L), WL3/4(L)
  DW1/1 -> WL/2(User)
  P1W2/1 -> WL1/2(User)

== system c00023M_harness/M167/Physical ==
  InW1 : Inport
  InW2 : Inport  Port=2
  InW3 : Inport  Port=3
  InW4 : Inport  Port=4
  W : Subsystem
  W5 : Subsystem
  W6 : Subsystem
  W7 : Subsystem
  W1 : Outport
  W2 : Outport  Port=2
  W3 : Outport  Port=3
  W4 : Outport  Port=4
  wires:
  W7/1(WPos) -> W4/1
  W6/1(WPos) -> W3/1
  W5/1(WPos) -> W2/1
  W/1(WPos) -> W1/1
  InW4/1 -> W7/1(WIn)
  InW3/1 -> W6/1(WIn)
  InW2/1 -> W5/1(WIn)
  InW1/1 -> W/1(WIn)

== system c00023M_harness/M167/S1 ==
  PhyMeasure : Inport
  SensorOut : Outport
  wires:
  PhyMeasure/1 -> SensorOut/1

== system c00023M_harness/M167/S2 ==
  PhyMeasure : Inport
  SensorOut : Outport
  wires:
  PhyMeasure/1 -> SensorOut/1

== system c00023M_harness/M167/S3 ==
  PhyMeasure : Inport
  SensorOut : Outport
  wires:
  PhyMeasure/1 -> SensorOut/1

== system c00023M_harness/M167/S4 ==
  PhyMeasure : Inport
  SensorOut : Outport
  wires:
  PhyMeasure/1 -> SensorOut/1

== system c00023M_harness/M168/Cyber ==
  note: Sensors
  note: Inputs For Window1
  note: Inputs for Window 2
  note: Inputs for window 3
  note: Inputs for window 4
  note: Users
  note: Users
  note: Sensors
  note: Users
  note: Sensors
  note: Users
  note: Sensors
  note: USERS
      | ---------------------------------
      | 0: None
      | 1: Ventana Arriba
      | 2: Ventana hasta arriba
      | 3: Ventana abajo
      | 4: Ventana hasta abajo
  note: 1: SUBE
      | 0: PARADO
      | -1 BAJA
  note: D = Driver (W1)
      | P1 = Passenger 1 (W2)
      | P2 = Passenger 2 (W3)
      | P3 = Passenger 3 (W4)
      | O = Obstacle
      | C = Control
      | Pri = Prioritizer
      | LD = LockDriver
      | PosW = PositionWindow
      | WL = WindowLogic
      | OW = ObstacleWindow
      | CWXC = ControlWindowXCentralized
      | S = Sensor
      | L = Lock
      | WPos = WindowPosition
      | M = Memory
      | InW = InputWindow
      | WIn = WindowInput
  PosW1 : Inport
  PosW2 : Inport  Port=2
  PosW3 : Inport  Port=3
  PosW4 : Inport  Port=4
  DW1 : Inport  Port=5
  DW3 : Inport  Port=6
  P1W2 : Inport  Port=7
  P2W3 : Inport  Port=8
  P3W4 : Inport  Port=9
  P1W4 : Inport  Port=10
  OW1 : Inport  Port=11
  OW2 : Inport  Port=12
  OW3 : Inport  Port=13
  OW4 : Inport  Port=14
  LD : Inport  Port=15
  CW3C : Inport  Port=16
  CW4C : Inport  Port=17
  Pri1 : Subsystem
  Pri4 : Subsystem
  WL : Subsystem
  WL1 : Subsystem
  WL2 : Subsystem
  WL3 : Subsystem
  W1 : Outport
  W2 : Outport  Port=2
  W3 : Outport  Port=3
  W4 : Outport  Port=4
  wires:
  CW4C/1 -> Pri4/3(CW4C)
  CW3C/1 -> Pri1/3(CW3C)
  WL3/1(WindowLogicOutput) -> W4/1
  WL2/1(WindowLogicOutput) -> W3/1
  Pri4/1(User) -> WL3/2(User)
  OW4/1 -> WL3/3(OW)
  PosW4/1 -> WL3/1(WPos)
  P1W4/1 -> Pri4/2(P1)
  P3W4/1 -> Pri4/1(P)
  P2W3/1 -> Pri1/2(P)
  DW3/1 -> Pri1/1(D)
  OW3/1 -> WL2/3(OW)
  PosW3/1 -> WL2/1(WPos)
  Pri1/1(User) -> WL2/2(User)
  WL1/1(WindowLogicOutput) -> W2/1
  OW2/1 -> WL1/3(OW)
  PosW2/1 -> WL1/1(WPos)
  WL/1(WindowLogicOutput) -> W1/1
  OW1/1 -> WL/3(OW)
  PosW1/1 -> WL/1(WPos)
  LD/1 -> WL2/4(L), WL3/4(L)
  DW1/1 -> WL/2(User)
  P1W2/1 -> WL1/2(User)

== system c00023M_harness/M168/Physical ==
  InW1 : Inport
  InW2 : Inport  Port=2
  InW3 : Inport  Port=3
  InW4 : Inport  Port=4
  W : Subsystem
  W5 : Subsystem
  W6 : Subsystem
  W7 : Subsystem
  W1 : Outport
  W2 : Outport  Port=2
  W3 : Outport  Port=3
  W4 : Outport  Port=4
  wires:
  W7/1(WPos) -> W4/1
  W6/1(WPos) -> W3/1
  W5/1(WPos) -> W2/1
  W/1(WPos) -> W1/1
  InW4/1 -> W7/1(WIn)
  InW3/1 -> W6/1(WIn)
  InW2/1 -> W5/1(WIn)
  InW1/1 -> W/1(WIn)

== system c00023M_harness/M168/S1 ==
  PhyMeasure : Inport
  SensorOut : Outport
  wires:
  PhyMeasure/1 -> SensorOut/1

== system c00023M_harness/M168/S2 ==
  PhyMeasure : Inport
  SensorOut : Outport
  wires:
  PhyMeasure/1 -> SensorOut/1

== system c00023M_harness/M168/S3 ==
  PhyMeasure : Inport
  SensorOut : Outport
  wires:
  PhyMeasure/1 -> SensorOut/1

== system c00023M_harness/M168/S4 ==
  PhyMeasure : Inport
  SensorOut : Outport
  wires:
  PhyMeasure/1 -> SensorOut/1

== system c00023M_harness/M169/Cyber ==
  note: Sensors
  note: Inputs For Window1
  note: Inputs for Window 2
  note: Inputs for window 3
  note: Inputs for window 4
  note: Users
  note: Users
  note: Sensors
  note: Users
  note: Sensors
  note: Users
  note: Sensors
  note: USERS
      | ---------------------------------
      | 0: None
      | 1: Ventana Arriba
      | 2: Ventana hasta arriba
      | 3: Ventana abajo
      | 4: Ventana hasta abajo
  note: 1: SUBE
      | 0: PARADO
      | -1 BAJA
  note: D = Driver (W1)
      | P1 = Passenger 1 (W2)
      | P2 = Passenger 2 (W3)
      | P3 = Passenger 3 (W4)
      | O = Obstacle
      | C = Control
      | Pri = Prioritizer
      | LD = LockDriver
      | PosW = PositionWindow
      | WL = WindowLogic
      | OW = ObstacleWindow
      | CWXC = ControlWindowXCentralized
      | S = Sensor
      | L = Lock
      | WPos = WindowPosition
      | M = Memory
      | InW = InputWindow
      | WIn = WindowInput
  PosW1 : Inport
  PosW2 : Inport  Port=2
  PosW3 : Inport  Port=3
  PosW4 : Inport  Port=4
  DW1 : Inport  Port=5
  DW3 : Inport  Port=6
  P1W2 : Inport  Port=7
  P2W3 : Inport  Port=8
  P3W4 : Inport  Port=9
  P1W4 : Inport  Port=10
  OW1 : Inport  Port=11
  OW2 : Inport  Port=12
  OW3 : Inport  Port=13
  OW4 : Inport  Port=14
  LD : Inport  Port=15
  CW3C : Inport  Port=16
  CW4C : Inport  Port=17
  Pri1 : Subsystem
  Pri4 : Subsystem
  WL : Subsystem
  WL1 : Subsystem
  WL2 : Subsystem
  WL3 : Subsystem
  W1 : Outport
  W2 : Outport  Port=2
  W3 : Outport  Port=3
  W4 : Outport  Port=4
  wires:
  CW4C/1 -> Pri4/3(CW4C)
  CW3C/1 -> Pri1/3(CW3C)
  WL3/1(WindowLogicOutput) -> W4/1
  WL2/1(WindowLogicOutput) -> W3/1
  Pri4/1(User) -> WL3/2(User)
  OW4/1 -> WL3/3(OW)
  PosW4/1 -> WL3/1(WPos)
  P1W4/1 -> Pri4/2(P1)
  P3W4/1 -> Pri4/1(P)
  P2W3/1 -> Pri1/2(P)
  DW3/1 -> Pri1/1(D)
  OW3/1 -> WL2/3(OW)
  PosW3/1 -> WL2/1(WPos)
  Pri1/1(User) -> WL2/2(User)
  WL1/1(WindowLogicOutput) -> W2/1
  OW2/1 -> WL1/3(OW)
  PosW2/1 -> WL1/1(WPos)
  WL/1(WindowLogicOutput) -> W1/1
  OW1/1 -> WL/3(OW)
  PosW1/1 -> WL/1(WPos)
  LD/1 -> WL2/4(L), WL3/4(L)
  DW1/1 -> WL/2(User)
  P1W2/1 -> WL1/2(User)

== system c00023M_harness/M169/Physical ==
  InW1 : Inport
  InW2 : Inport  Port=2
  InW3 : Inport  Port=3
  InW4 : Inport  Port=4
  W : Subsystem
  W5 : Subsystem
  W6 : Subsystem
  W7 : Subsystem
  W1 : Outport
  W2 : Outport  Port=2
  W3 : Outport  Port=3
  W4 : Outport  Port=4
  wires:
  W7/1(WPos) -> W4/1
  W6/1(WPos) -> W3/1
  W5/1(WPos) -> W2/1
  W/1(WPos) -> W1/1
  InW4/1 -> W7/1(WIn)
  InW3/1 -> W6/1(WIn)
  InW2/1 -> W5/1(WIn)
  InW1/1 -> W/1(WIn)

== system c00023M_harness/M169/S1 ==
  PhyMeasure : Inport
  SensorOut : Outport
  wires:
  PhyMeasure/1 -> SensorOut/1

== system c00023M_harness/M169/S2 ==
  PhyMeasure : Inport
  SensorOut : Outport
  wires:
  PhyMeasure/1 -> SensorOut/1

== system c00023M_harness/M169/S3 ==
  PhyMeasure : Inport
  SensorOut : Outport
  wires:
  PhyMeasure/1 -> SensorOut/1

== system c00023M_harness/M169/S4 ==
  PhyMeasure : Inport
  SensorOut : Outport
  wires:
  PhyMeasure/1 -> SensorOut/1

== system c00023M_harness/M170/Cyber ==
  note: Sensors
  note: Inputs For Window1
  note: Inputs for Window 2
  note: Inputs for window 3
  note: Inputs for window 4
  note: Users
  note: Users
  note: Sensors
  note: Users
  note: Sensors
  note: Users
  note: Sensors
  note: USERS
      | ---------------------------------
      | 0: None
      | 1: Ventana Arriba
      | 2: Ventana hasta arriba
      | 3: Ventana abajo
      | 4: Ventana hasta abajo
  note: 1: SUBE
      | 0: PARADO
      | -1 BAJA
  note: D = Driver (W1)
      | P1 = Passenger 1 (W2)
      | P2 = Passenger 2 (W3)
      | P3 = Passenger 3 (W4)
      | O = Obstacle
      | C = Control
      | Pri = Prioritizer
      | LD = LockDriver
      | PosW = PositionWindow
      | WL = WindowLogic
      | OW = ObstacleWindow
      | CWXC = ControlWindowXCentralized
      | S = Sensor
      | L = Lock
      | WPos = WindowPosition
      | M = Memory
      | InW = InputWindow
      | WIn = WindowInput
  PosW1 : Inport
  PosW2 : Inport  Port=2
  PosW3 : Inport  Port=3
  PosW4 : Inport  Port=4
  DW1 : Inport  Port=5
  DW3 : Inport  Port=6
  P1W2 : Inport  Port=7
  P2W3 : Inport  Port=8
  P3W4 : Inport  Port=9
  P1W4 : Inport  Port=10
  OW1 : Inport  Port=11
  OW2 : Inport  Port=12
  OW3 : Inport  Port=13
  OW4 : Inport  Port=14
  LD : Inport  Port=15
  CW3C : Inport  Port=16
  CW4C : Inport  Port=17
  Pri1 : Subsystem
  Pri4 : Subsystem
  WL : Subsystem
  WL1 : Subsystem
  WL2 : Subsystem
  WL3 : Subsystem
  W1 : Outport
  W2 : Outport  Port=2
  W3 : Outport  Port=3
  W4 : Outport  Port=4
  wires:
  CW4C/1 -> Pri4/3(CW4C)
  CW3C/1 -> Pri1/3(CW3C)
  WL3/1(WindowLogicOutput) -> W4/1
  WL2/1(WindowLogicOutput) -> W3/1
  Pri4/1(User) -> WL3/2(User)
  OW4/1 -> WL3/3(OW)
  PosW4/1 -> WL3/1(WPos)
  P1W4/1 -> Pri4/2(P1)
  P3W4/1 -> Pri4/1(P)
  P2W3/1 -> Pri1/2(P)
  DW3/1 -> Pri1/1(D)
  OW3/1 -> WL2/3(OW)
  PosW3/1 -> WL2/1(WPos)
  Pri1/1(User) -> WL2/2(User)
  WL1/1(WindowLogicOutput) -> W2/1
  OW2/1 -> WL1/3(OW)
  PosW2/1 -> WL1/1(WPos)
  WL/1(WindowLogicOutput) -> W1/1
  OW1/1 -> WL/3(OW)
  PosW1/1 -> WL/1(WPos)
  LD/1 -> WL2/4(L), WL3/4(L)
  DW1/1 -> WL/2(User)
  P1W2/1 -> WL1/2(User)

== system c00023M_harness/M170/Physical ==
  InW1 : Inport
  InW2 : Inport  Port=2
  InW3 : Inport  Port=3
  InW4 : Inport  Port=4
  W : Subsystem
  W5 : Subsystem
  W6 : Subsystem
  W7 : Subsystem
  W1 : Outport
  W2 : Outport  Port=2
  W3 : Outport  Port=3
  W4 : Outport  Port=4
  wires:
  W7/1(WPos) -> W4/1
  W6/1(WPos) -> W3/1
  W5/1(WPos) -> W2/1
  W/1(WPos) -> W1/1
  InW4/1 -> W7/1(WIn)
  InW3/1 -> W6/1(WIn)
  InW2/1 -> W5/1(WIn)
  InW1/1 -> W/1(WIn)

== system c00023M_harness/M170/S1 ==
  PhyMeasure : Inport
  SensorOut : Outport
  wires:
  PhyMeasure/1 -> SensorOut/1

== system c00023M_harness/M170/S2 ==
  PhyMeasure : Inport
  SensorOut : Outport
  wires:
  PhyMeasure/1 -> SensorOut/1

== system c00023M_harness/M170/S3 ==
  PhyMeasure : Inport
  SensorOut : Outport
  wires:
  PhyMeasure/1 -> SensorOut/1

== system c00023M_harness/M170/S4 ==
  PhyMeasure : Inport
  SensorOut : Outport
  wires:
  PhyMeasure/1 -> SensorOut/1

== system c00023M_harness/M171/Cyber ==
  note: Sensors
  note: Inputs For Window1
  note: Inputs for Window 2
  note: Inputs for window 3
  note: Inputs for window 4
  note: Users
  note: Users
  note: Sensors
  note: Users
  note: Sensors
  note: Users
  note: Sensors
  note: USERS
      | ---------------------------------
      | 0: None
      | 1: Ventana Arriba
      | 2: Ventana hasta arriba
      | 3: Ventana abajo
      | 4: Ventana hasta abajo
  note: 1: SUBE
      | 0: PARADO
      | -1 BAJA
  note: D = Driver (W1)
      | P1 = Passenger 1 (W2)
      | P2 = Passenger 2 (W3)
      | P3 = Passenger 3 (W4)
      | O = Obstacle
      | C = Control
      | Pri = Prioritizer
      | LD = LockDriver
      | PosW = PositionWindow
      | WL = WindowLogic
      | OW = ObstacleWindow
      | CWXC = ControlWindowXCentralized
      | S = Sensor
      | L = Lock
      | WPos = WindowPosition
      | M = Memory
      | InW = InputWindow
      | WIn = WindowInput
  PosW1 : Inport
  PosW2 : Inport  Port=2
  PosW3 : Inport  Port=3
  PosW4 : Inport  Port=4
  DW1 : Inport  Port=5
  DW3 : Inport  Port=6
  P1W2 : Inport  Port=7
  P2W3 : Inport  Port=8
  P3W4 : Inport  Port=9
  P1W4 : Inport  Port=10
  OW1 : Inport  Port=11
  OW2 : Inport  Port=12
  OW3 : Inport  Port=13
  OW4 : Inport  Port=14
  LD : Inport  Port=15
  CW3C : Inport  Port=16
  CW4C : Inport  Port=17
  Pri1 : Subsystem
  Pri4 : Subsystem
  WL : Subsystem
  WL1 : Subsystem
  WL2 : Subsystem
  WL3 : Subsystem
  W1 : Outport
  W2 : Outport  Port=2
  W3 : Outport  Port=3
  W4 : Outport  Port=4
  wires:
  CW4C/1 -> Pri4/3(CW4C)
  CW3C/1 -> Pri1/3(CW3C)
  WL3/1(WindowLogicOutput) -> W4/1
  WL2/1(WindowLogicOutput) -> W3/1
  Pri4/1(User) -> WL3/2(User)
  OW4/1 -> WL3/3(OW)
  PosW4/1 -> WL3/1(WPos)
  P1W4/1 -> Pri4/2(P1)
  P3W4/1 -> Pri4/1(P)
  P2W3/1 -> Pri1/2(P)
  DW3/1 -> Pri1/1(D)
  OW3/1 -> WL2/3(OW)
  PosW3/1 -> WL2/1(WPos)
  Pri1/1(User) -> WL2/2(User)
  WL1/1(WindowLogicOutput) -> W2/1
  OW2/1 -> WL1/3(OW)
  PosW2/1 -> WL1/1(WPos)
  WL/1(WindowLogicOutput) -> W1/1
  OW1/1 -> WL/3(OW)
  PosW1/1 -> WL/1(WPos)
  LD/1 -> WL2/4(L), WL3/4(L)
  DW1/1 -> WL/2(User)
  P1W2/1 -> WL1/2(User)

== system c00023M_harness/M171/Physical ==
  InW1 : Inport
  InW2 : Inport  Port=2
  InW3 : Inport  Port=3
  InW4 : Inport  Port=4
  W : Subsystem
  W5 : Subsystem
  W6 : Subsystem
  W7 : Subsystem
  W1 : Outport
  W2 : Outport  Port=2
  W3 : Outport  Port=3
  W4 : Outport  Port=4
  wires:
  W7/1(WPos) -> W4/1
  W6/1(WPos) -> W3/1
  W5/1(WPos) -> W2/1
  W/1(WPos) -> W1/1
  InW4/1 -> W7/1(WIn)
  InW3/1 -> W6/1(WIn)
  InW2/1 -> W5/1(WIn)
  InW1/1 -> W/1(WIn)

== system c00023M_harness/M171/S1 ==
  PhyMeasure : Inport
  SensorOut : Outport
  wires:
  PhyMeasure/1 -> SensorOut/1

== system c00023M_harness/M171/S2 ==
  PhyMeasure : Inport
  SensorOut : Outport
  wires:
  PhyMeasure/1 -> SensorOut/1
